simulink subsystem "Orbit_sim"  (R2024a)
settings: Solver=VariableStepAuto  StartTime=0.0  StopTime=10.0  RelTol=1e-3
undefined symbols (not defined in the file or in its folder): J1, J2, J3
settings Model: Creator=ruimi  LastModifiedBy=alenachan

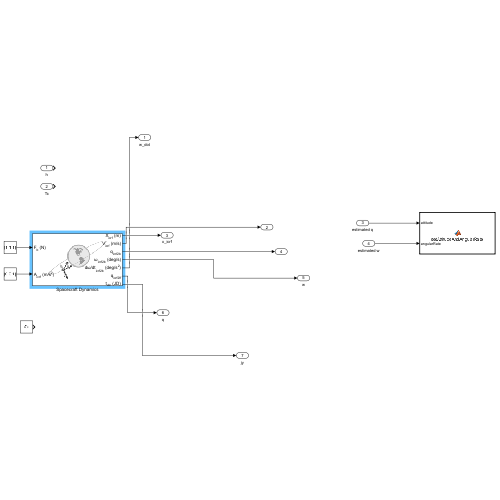
[thumbnail: Simulink's stored preview of the top-level diagram]
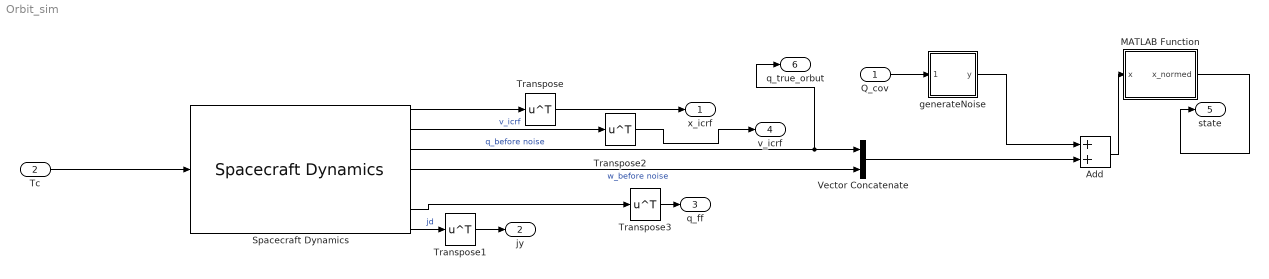
== system Orbit_sim ==
  Q_cov : Inport
  Tc : Inport  Port=2
  Add : Sum
  MATLAB Function : MATLAB Function  TreatAsAtomicUnit=on
  Spacecraft Dynamics : SpacecraftDynamics  forcesIn=off  startDate=2458850.00000058  mass=m  inertia=[J1,0,0;0,J2,0;0,0,J3]  stateFormatNum=ICRF state vector  semiMajorAxis=6789000  eccentricity=0.001  inclination=Orbit_Incl  raan=299.4750  argPeriapsis=347.2333  trueAnomaly=109  inertialPosition=[3649699.96179444 3308200.09258889 -4676599.96425833]  inertialVelocity=[-2750.7999951343 6666.40000211443 2573.40000744743]  attitudeFrame=NED  attitude=[-0.111705467945673 -0.70150298408038 -0.0584495584026014 0.701426475747745]  attitudeRate=[-148025.938056461 -259659.807922711 192872.307113357]  outputAngAccel=on  earthSH=EGM96  outputTransform=on  useDrag=on  useSRP=on  units=Metric (km/h)
  Transpose{,1..3} (4 alike) : Math  Operator=transpose
  Vector Concatenate : Concatenate
  generateNoise : MATLAB Function  Priority=1  TreatAsAtomicUnit=on
  x_icrf : Outport
  jy : Outport  Port=2
  q_ff : Outport  Port=3
  v_icrf : Outport  Port=4
  state : Outport  Port=5
  q_true_orbut : Outport  Port=6
  wires:
  Spacecraft Dynamics/4 -> Vector Concatenate/2  "w_before noise"
  Spacecraft Dynamics/7 -> Transpose1/1  "jd"
  Spacecraft Dynamics/1 -> Transpose/1
  Tc/1 -> Spacecraft Dynamics/1
  Spacecraft Dynamics/3 -> q_true_orbut/1, Vector Concatenate/1  "q_before noise"
  Transpose/1 -> x_icrf/1
  Transpose1/1 -> jy/1
  Spacecraft Dynamics/6 -> Transpose3/1
  Spacecraft Dynamics/2 -> Transpose2/1  "v_icrf"
  Transpose2/1 -> v_icrf/1
  Transpose3/1 -> q_ff/1
  Vector Concatenate/1 -> Add/2
  generateNoise/1(y) -> Add/1
  Q_cov/1 -> generateNoise/1(Sigma)
  Add/1 -> MATLAB Function/1(x)
  MATLAB Function/1(x_normed) -> state/1

== matlab function Orbit_sim/MATLAB Function ==
  data: x input; x_normed output
function x_normed = fcn(x)
x_normed = zeros(7,1);
x_normed(1:4) = x(1:4)/norm(x(1:4));
x_normed(5:7) = x(5:7);

== matlab function Orbit_sim/generateNoise ==
  data: y output; Sigma input
function y = Noise(Sigma)
secs = mod(mod(now,1)*1000000, 1000);
rng(secs);
mu = [0 0 0 0 0 0 0] ; %mean is zero for noise
%covariance is constant throughout, we take the input
y_temp = mvnrnd(mu,Sigma,1);
y = transpose(y_temp);
end
